simulink model "model"  (R2020b)
settings: Solver=VariableStepAuto  StartTime=0.0  StopTime=10.0  RelTol=1e-3
undefined symbols (not defined in the file): b, k1, k12, M1, M2
settings Model: Creator=Vrunda M Balgi  LastModifiedBy=Vrunda M Balgi

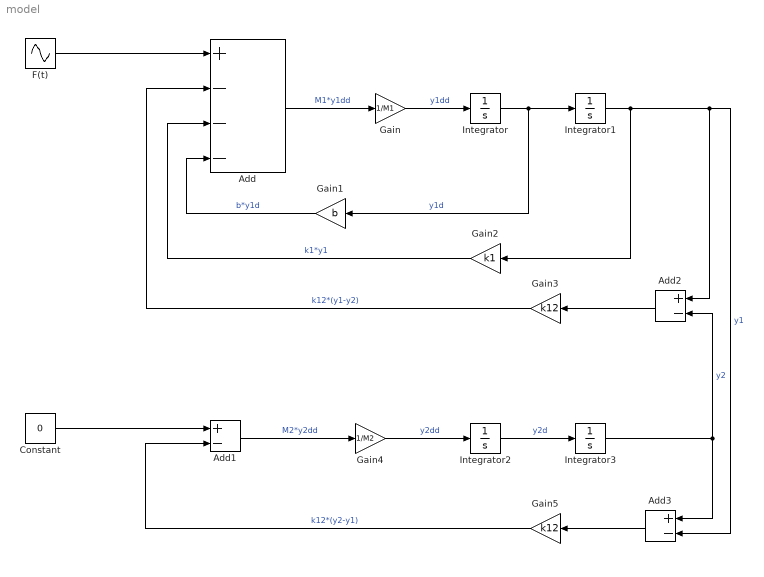
== system model ==
  Add : Sum  Inputs=+---
  Add1 : Sum  Inputs=+-
  Add2 : Sum  Inputs=+-
  Add3 : Sum  Inputs=+-
  Constant : Constant  Value=0
  F(t) : Sin  Amplitude=2  Frequency=10  SampleTime=0
  Gain : Gain  Gain=1/M1
  Gain1 : Gain  Gain=b
  Gain2 : Gain  Gain=k1
  Gain3 : Gain  Gain=k12
  Gain4 : Gain  Gain=1/M2
  Gain5 : Gain  Gain=k12
  Integrator{,1..3} (4 alike) : Integrator
  wires:
  Add/1 -> Gain/1  "M1*y1dd"
  Gain/1 -> Integrator/1  "y1dd"
  Integrator/1 -> Gain1/1, Integrator1/1  "y1d"
  Integrator1/1 -> Add2/1, Add3/2, Gain2/1  "y1"
  F(t)/1 -> Add/1
  Gain1/1 -> Add/4  "b*y1d"
  Gain2/1 -> Add/3  "k1*y1"
  Gain3/1 -> Add/2  "k12*(y1-y2)"
  Integrator2/1 -> Integrator3/1  "y2d"
  Integrator3/1 -> Add3/1, Add2/2  "y2"
  Gain4/1 -> Integrator2/1  "y2dd"
  Add1/1 -> Gain4/1  "M2*y2dd"
  Add2/1 -> Gain3/1
  Add3/1 -> Gain5/1
  Gain5/1 -> Add1/2  "k12*(y2-y1)"
  Constant/1 -> Add1/1
